simulink library "rad"  (Simulink 8.1)
settings: Solver=ode1  StartTime=0.0  StopTime=Inf  FixedStep=0.001  RelTol=1e-3
PostLoadFcn:
  | , if any(exist('dsrtsu_mdlpostloadfcn', 'file') == [2, 3, 6]), try dsrtsu_mdlpostloadfcn('Execute', bdroot); catch fprintf('Error in PostLoadFcn (dsrtsu_mdlpostloadfcn) for model "%s":\n %s\n', bdroot, lasterr); end, end,
undefined symbols (not defined in the file or in its folder): ENUM_RADPOWER_HIGH, ENUM_RADRXMISSING_NONE, ENUM_SENSORSTATE_FAILURE, ENUM_SENSORSTATE_NORMAL
settings Model: DSRTSU_INTERNAL_RTI_VER=450  DSRTSU_INTERNAL_RTI_TYPE=rti1401  RTICANMMDATA=struct('GeneralSetupData',struct('modelroot','D:\PROJECTS\HAITEC\06_Working_files\Subversion\trunk\AdasDragon\software\sw_development\arch\app\per','generalsettings',struct('filesettings',struct('destfolder',struct('Name','RTICANMM_FILES','Check',1),'buildfolder',struct('Name','.','Check',1),'AbsDestfolder',struct('Name','D:\PROJECTS\HAITEC\06_Working_files\Subversion\trunk\AdasDragon\software\sw_development\arch\app\per\RTICANMM_FILES'),'AbsBuildfolder',struct('Name','D:\PROJECTS\HAITEC\06_Working_files\Subversion\trunk\AdasDragon\software\sw_development\arch\app\per'))),'options',struct('addpaths',1,'rmpaths',1,'addtrcexclusion',logical(1),'cannavigator',struct('checkmonitoring',0),'show_usrtrc',0,'use_usrtrc',0),'advanced',struct('options',[1 1 1 1 1 1 1 1 1 1 1 1 1 1 1 1 1 1 1 1 1 1 1 1 1 1 1 1 1 1 1 1 1 1 1 1 1 1 1 1 1 1 1 1 1 1 1 1 1 1 1 1 1 1 1 1 1 1 1 1 1 1 1 1 1 1 1 1 1 1 1 1 1 1 1 1 1 1 1 1 1 1 1 1 1 1 1 1 1 1 1 1 1 1 1 1 1 1 1 1]),'MPSetup',{{}},'modelname','rad','block','rad'))  DSRTSU_INTERNAL_RTIFPGA=40  Creator=tescamilla  LastModifiedBy=tescamilla

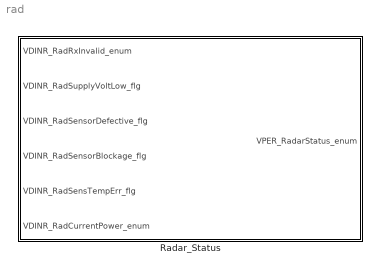
== system rad ==
  Radar_Status : Subsystem

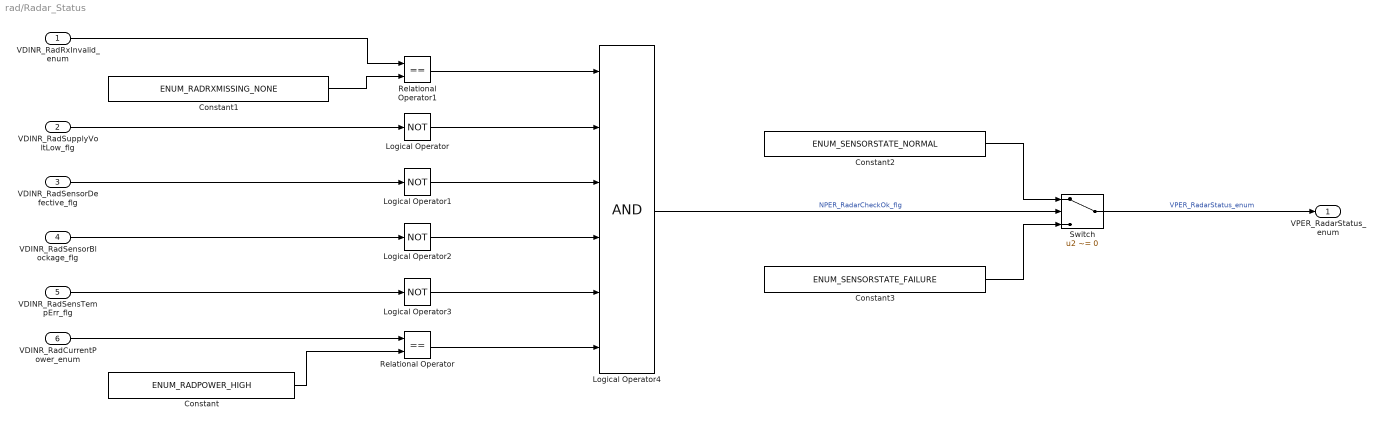
== system rad/Radar_Status ==
  VDINR_RadRxInvalid_enum : Inport
  VDINR_RadSupplyVoltLow_flg : Inport  Port=2
  VDINR_RadSensorDefective_flg : Inport  Port=3
  VDINR_RadSensorBlockage_flg : Inport  Port=4
  VDINR_RadSensTempErr_flg : Inport  Port=5
  VDINR_RadCurrentPower_enum : Inport  Port=6
  Constant : Constant  Value=ENUM_RADPOWER_HIGH
  Constant1 : Constant  Value=ENUM_RADRXMISSING_NONE
  Constant2 : Constant  Value=ENUM_SENSORSTATE_NORMAL
  Constant3 : Constant  Value=ENUM_SENSORSTATE_FAILURE
  Logical Operator{,1..3} (4 alike) : Logic  Operator=NOT  AllPortsSameDT=off  OutDataTypeStr=boolean
  Logical Operator4 : Logic  Inputs=6  AllPortsSameDT=off  OutDataTypeStr=boolean
  Relational Operator : RelationalOperator  Operator===  OutDataTypeStr=boolean
  Relational Operator1 : RelationalOperator  Operator===  OutDataTypeStr=boolean
  Switch : Switch  Criteria=u2 ~= 0
  VPER_RadarStatus_enum : Outport
  wires:
  VDINR_RadCurrentPower_enum/1 -> Relational Operator/1
  Constant/1 -> Relational Operator/2
  VDINR_RadRxInvalid_enum/1 -> Relational Operator1/1
  Constant1/1 -> Relational Operator1/2
  VDINR_RadSupplyVoltLow_flg/1 -> Logical Operator/1
  VDINR_RadSensorDefective_flg/1 -> Logical Operator1/1
  VDINR_RadSensorBlockage_flg/1 -> Logical Operator2/1
  VDINR_RadSensTempErr_flg/1 -> Logical Operator3/1
  Relational Operator/1 -> Logical Operator4/6
  Logical Operator3/1 -> Logical Operator4/5
  Logical Operator2/1 -> Logical Operator4/4
  Logical Operator1/1 -> Logical Operator4/3
  Logical Operator/1 -> Logical Operator4/2
  Relational Operator1/1 -> Logical Operator4/1
  Logical Operator4/1 -> Switch/2  "NPER_RadarCheckOk_flg"
  Constant2/1 -> Switch/1
  Constant3/1 -> Switch/3
  Switch/1 -> VPER_RadarStatus_enum/1  "VPER_RadarStatus_enum"
